simulink model "test_onoff_button_completebehavior"  (R2022b)
settings: Solver=FixedStepAuto  StartTime=0.0  StopTime=240  FixedStep=0.1  RelTol=1e-3
settings Model: Creator=cristian  LastModifiedBy=cristian
settings ConfigComp: CovEnable=on  RecordCoverage=on  CovModelRefEnable=on

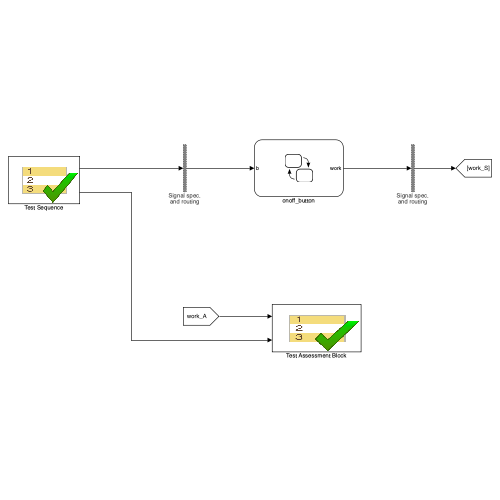
[thumbnail: Simulink's stored preview of the top-level diagram]
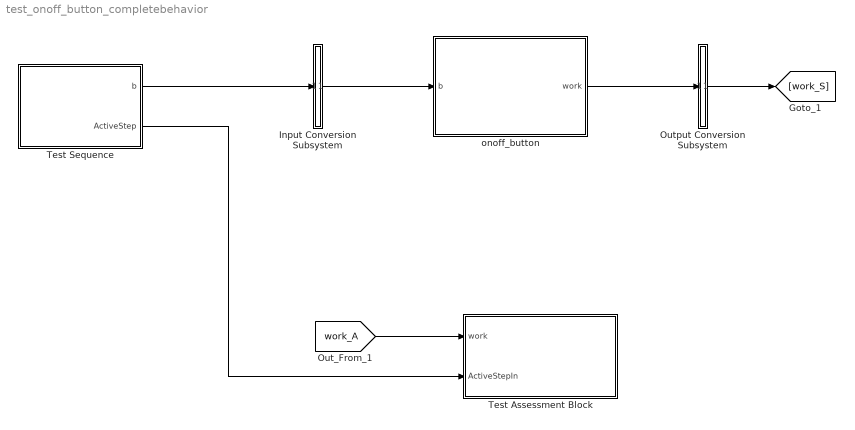
== system test_onoff_button_completebehavior ==
  Input Conversion Subsystem : Subsystem  Tag=__SLT_ICS__  Description=|
      | Signal spec.
      | and routing
      settings: AttributesFormatString=%<Description>
  Output Conversion Subsystem : Subsystem  Tag=__SLT_OCS__  Description=|
      | Signal spec.
      | and routing
      settings: AttributesFormatString=%<Description>
  Test Assessment Block : Test Sequence  Tag=__SLT_ASMT__  TreatAsAtomicUnit=on
  Test Sequence : Test Sequence  TreatAsAtomicUnit=on
  onoff_button : Stateflow chart  TreatAsAtomicUnit=on
  wires:
  Output Conversion Subsystem/1(Outport_1) -> [work_S]
  Input Conversion Subsystem/1(Outport_1) -> onoff_button/1(b)
  onoff_button/1(work) -> Output Conversion Subsystem/1(Inport_1)
  Test Sequence/1(b) -> Input Conversion Subsystem/1(Inport_1)
  Test Sequence/2(ActiveStep) -> Test Assessment Block/2(ActiveStepIn)
  [work_A] -> Test Assessment Block/1(work)

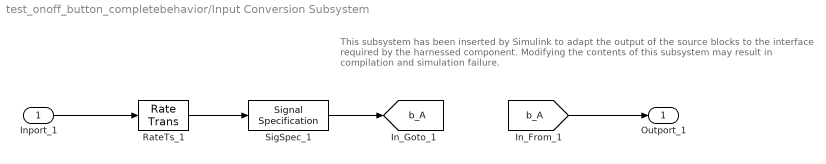
== system test_onoff_button_completebehavior/Input Conversion Subsystem ==
  note: This subsystem has been inserted by Simulink to adapt the output of the source blocks to the interface required by the harnessed component.
      |  Modifying the contents of this subsystem may result in compilation and simulation failure.
  Inport_1 : Inport
  RateTs_1 : RateTransition  OutPortSampleTime=[-1, 0]
  SigSpec_1 : SignalSpecification  OutDataTypeStr=boolean  Dimensions=[1]  SampleTime=[-1, 0]
  Outport_1 : Outport
  tag scope: b_A=global
  wires:
  [b_A] -> Outport_1/1
  SigSpec_1/1 -> [b_A]
  RateTs_1/1 -> SigSpec_1/1
  Inport_1/1 -> RateTs_1/1

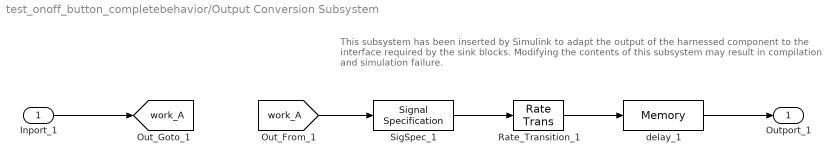
== system test_onoff_button_completebehavior/Output Conversion Subsystem ==
  note: This subsystem has been inserted by Simulink to adapt the output of the harnessed component to the interface required by the sink blocks.
      |  Modifying the contents of this subsystem may result in compilation and simulation failure.
  Inport_1 : Inport
  Rate_Transition_1 : RateTransition  OutPortSampleTimeOpt=Inherit
  SigSpec_1 : SignalSpecification  OutDataTypeStr=boolean  Dimensions=[1]
  delay_1 : Memory
  Outport_1 : Outport
  tag scope: work_A=global
  wires:
  Inport_1/1 -> [work_A]
  [work_A] -> SigSpec_1/1
  SigSpec_1/1 -> Rate_Transition_1/1
  Rate_Transition_1/1 -> delay_1/1
  delay_1/1 -> Outport_1/1

== stateflow chart test_onoff_button_completebehavior/Test Assessment Block ==
  state CompleteBehavior
    state Run
      state Verify_CB_Init
        verify(work == 0);
      state Verify_CB_Inactive_Wait
        verify(work == 0);
      state Verify_CB_Inactive_Pressed
        verify(work == 1);
      state Verify_CB_Active_Wait
        verify(work == 1);
      state Verify_CB_Active_Pressed
        verify(work == 1);
      state Verify_CB_Active_Released
        verify(work == 1);
      state Verify_CB_Active_PressedAgain
        verify(work == 1);
      state Verify_CB_Active_LongPressed
        verify(work == 1);
      state Verify_CB_Active_NoWork
        verify(work == 0);
      state Verify_CB_Backto_Inactive
        verify(work == 0);
      state Verify_CB_Void
      (default) -> (junction 180)
      Run -> (junction 180)
      (junction 180) -> (junction 181) [order 1] : [ActiveStepIn == ActiveStepEnumH2.CB_Init
          | ]
      (junction 181) -> Verify_CB_Init [order 1] : [~in(CompleteBehavior.Run.Verify_CB_Init)]
      (junction 180) -> (junction 189) [order 2]
      (junction 181) -> (junction 184) [order 2]
      (junction 189) -> (junction 190) [order 1] : [ActiveStepIn == ActiveStepEnumH2.CB_Inactive_Wait
          | ]
      (junction 190) -> Verify_CB_Inactive_Wait [order 1] : [~in(CompleteBehavior.Run.Verify_CB_Inactive_Wait)]
      (junction 189) -> (junction 252) [order 2]
      (junction 190) -> (junction 193) [order 2]
      (junction 252) -> (junction 253) [order 1] : [ActiveStepIn == ActiveStepEnumH2.CB_Inactive_Pressed
          | ]
      (junction 253) -> Verify_CB_Inactive_Pressed [order 1] : [~in(CompleteBehavior.Run.Verify_CB_Inactive_Pressed)]
      (junction 252) -> (junction 270) [order 2]
      (junction 253) -> (junction 256) [order 2]
      (junction 270) -> (junction 271) [order 1] : [ActiveStepIn == ActiveStepEnumH2.CB_Active_Wait
          | ]
      (junction 271) -> Verify_CB_Active_Wait [order 1] : [~in(CompleteBehavior.Run.Verify_CB_Active_Wait)]
      (junction 270) -> (junction 288) [order 2]
      (junction 271) -> (junction 274) [order 2]
      (junction 288) -> (junction 289) [order 1] : [ActiveStepIn == ActiveStepEnumH2.CB_Active_Pressed
          | ]
      (junction 289) -> Verify_CB_Active_Pressed [order 1] : [~in(CompleteBehavior.Run.Verify_CB_Active_Pressed)]
      (junction 288) -> (junction 297) [order 2]
      (junction 289) -> (junction 292) [order 2]
      (junction 297) -> (junction 298) [order 1] : [ActiveStepIn == ActiveStepEnumH2.CB_Active_Released
          | ]
      (junction 298) -> Verify_CB_Active_Released [order 1] : [~in(CompleteBehavior.Run.Verify_CB_Active_Released)]
      (junction 297) -> (junction 306) [order 2]
      (junction 298) -> (junction 301) [order 2]
      (junction 306) -> (junction 307) [order 1] : [ActiveStepIn == ActiveStepEnumH2.CB_Active_PressedAgain
          | ]
      (junction 307) -> Verify_CB_Active_PressedAgain [order 1] : [~in(CompleteBehavior.Run.Verify_CB_Active_PressedAgain)]
      (junction 306) -> (junction 315) [order 2]
      (junction 307) -> (junction 310) [order 2]
      (junction 315) -> (junction 316) [order 1] : [ActiveStepIn == ActiveStepEnumH2.CB_Active_LongPressed
          | ]
      (junction 316) -> Verify_CB_Active_LongPressed [order 1] : [~in(CompleteBehavior.Run.Verify_CB_Active_LongPressed)]
      (junction 345) -> (junction 333) [order 2]
      (junction 316) -> (junction 319) [order 2]
      (junction 345) -> (junction 346) [order 1] : [ActiveStepIn == ActiveStepEnumH2.CB_Active_NoWork
          | ]
      (junction 346) -> Verify_CB_Active_NoWork [order 1] : [~in(CompleteBehavior.Run.Verify_CB_Active_NoWork)]
      (junction 333) -> (junction 334) [order 1] : [ActiveStepIn == ActiveStepEnumH2.CB_Backto_Inactive
          | ]
      (junction 334) -> Verify_CB_Backto_Inactive [order 1] : [~in(CompleteBehavior.Run.Verify_CB_Backto_Inactive)]
      (junction 333) -> (junction 260) [order 2]
      (junction 334) -> (junction 337) [order 2]
      (junction 260) -> (junction 261)
      (junction 261) -> Verify_CB_Void [order 1] : [~in(CompleteBehavior.Run.Verify_CB_Void)]
      (junction 261) -> (junction 264) [order 2]
      (junction 346) -> (junction 349) [order 2]
      (junction 315) -> (junction 345) [order 2]
    (default) -> Run
  (default) -> CompleteBehavior : {assert(Active_Scenario_Index == 1,'The value of Scenario Parameter ''Active_Scenario_Index'' is not valid. Use the index of the scenario to specify it.')}
  data: work input boolean size=[1]; ActiveStepIn input; Active_Scenario_Index parameter =1

== stateflow chart test_onoff_button_completebehavior/onoff_button ==
  note: Stato di accensione del bottone onoff
  note: In questo stato il bottone può accendere la macchina
  state INACTIVE
    state Pressed
      en: work = HIGH
    state Wait
      en: work = LOW
    (default) -> INACTIVE.Wait
    INACTIVE.Wait -> INACTIVE.Pressed : [b == PRESSED]
  note: Stato di spegnimento del bottone onoff
  note: In questo stato il bottone può spengere la macchina
  state ACTIVE
    state Wait
      en:
      b_long = RELEASED
    state Pressed
      en:
      b_long = RELEASED;
      on after(DURATION,sec): b_long = PRESSED
    state LongPressed
      en: work = LOW;
    (default) -> ACTIVE.Wait
    ACTIVE.Wait -> ACTIVE.Pressed : [b == PRESSED]
    ACTIVE.Pressed -> ACTIVE.Wait [order 1] : [b == RELEASED]
    ACTIVE.Pressed -> LongPressed [order 2] : [b_long == PRESSED && b == PRESSED]
  note: Se il bottone viene premuto una sola volta, il sistema viene acceso.
      | Se il bottone viene premuto per 1 secondo, il sistema viene spento.
      | Una pressione prolungata senza rilascio del bottone, non causa un alternarsi di accensioni e spegnimenti continui.
  (default) -> INACTIVE
  INACTIVE.Pressed -> ACTIVE : [b == RELEASED]
  LongPressed -> INACTIVE : [b==RELEASED]
  data: PRESSED constant boolean size=1 =0; RELEASED constant boolean size=1 =1; b input boolean size=1; DURATION constant double size=1 =1; b_long local boolean size=1; HIGH constant boolean size=1 =1; LOW constant boolean size=1 =0; work output boolean size=1

== stateflow chart test_onoff_button_completebehavior/Test Sequence ==
  settings: updateMethod=DISCRETE  sampleTime=0.1
  state CompleteBehavior
    state CB_Init
      b = true
      settings: description=Partiamo da uno stato in cui il bottone non è premuto.
    state CB_Inactive_Wait
      b = true
    state CB_Inactive_Pressed
      b = false
      settings: description=Effettuiamo la pressione del bottone per dare il segnale di work alto
    state CB_Active_Wait
      b = true
      settings: description=Rilasciamo il bottone, mi aspetto che il modello si predisponga per comportarsi come un bottone a livelli.
    state CB_Active_Pressed
      b = false
      settings: description=Premiamo di nuovo
    state CB_Active_Released
      b = true
      settings: description=Rilasciamo senza dare il tempo di fare impostare il livello del bottone
    state CB_Active_PressedAgain
      b  = false
      settings: description=premiamo il bottone
    state CB_Active_LongPressed
      b = false
      settings: description=Manteniamo la pressione per un secondo
    state CB_Active_NoWork
      b = false
      settings: description=Mi aspetto di avere un segnale work = false, ovvero il sistema dovrebbe ricevere l'input di spegnersi
    state CB_Backto_Inactive
      b = true
      settings: description=Rilascio definitivamente
    (default) -> CB_Init
    CB_Init -> CB_Inactive_Wait : [
        | true
        | ]
    CB_Inactive_Wait -> CB_Inactive_Pressed : [
        | true
        | ]
    CB_Inactive_Pressed -> CB_Active_Wait : [
        | true
        | ]
    CB_Active_Wait -> CB_Active_Pressed : [
        | true
        | ]
    CB_Active_Pressed -> CB_Active_Released : [
        | true
        | ]
    CB_Active_Released -> CB_Active_PressedAgain : [
        | true
        | ]
    CB_Active_PressedAgain -> CB_Active_LongPressed : [
        | true
        | ]
    CB_Active_LongPressed -> CB_Active_NoWork : [
        | after(1,sec)
        | ]
    CB_Active_NoWork -> CB_Backto_Inactive : [
        | true
        | ]
  (default) -> CompleteBehavior : {assert(Active_Scenario_Index == 1,'The value of Scenario Parameter ''Active_Scenario_Index'' is not valid. Use the index of the scenario to specify it.')}
  data: b output boolean size=[1]; Active_Scenario_Index parameter =1; ActiveStep output Enum: ActiveStepEnumH2; sample_time constant double =str2num(get_param('InductionCooker','FixedStep'))
